simulink model "EKF_MDL"  (R2013a)
settings: Solver=VariableStepDiscrete  StartTime=0.0  StopTime=50  RelTol=1e-3
settings Model: Creator=Aleksandr  LastModifiedBy=Aleksandr

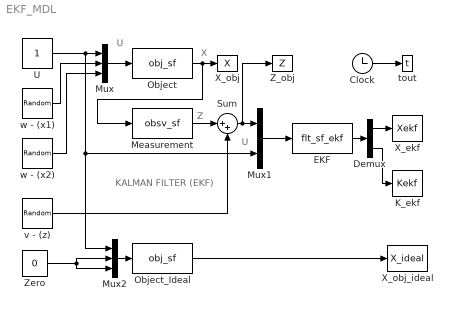
== system EKF_MDL ==
  note: KALMAN FILTER
      | (EKF)
  note: U
  note: Z
  note: U
  note: X
  Clock : Clock
      settings: Decimation=100
  Demux : Demux  Outputs=2
  EKF : S-Function  FunctionName=flt_sf_ekf  EnableBusSupport=off
  K_ekf : ToWorkspace  VariableName=Kekf  SampleTime=-1
  Measurement : S-Function  FunctionName=obsv_sf  EnableBusSupport=off
  Mux : Mux  Inputs=3
  Mux1 : Mux  Inputs=2
  Mux2 : Mux  Inputs=3
  Object : S-Function  FunctionName=obj_sf  EnableBusSupport=off
  Object_Ideal : S-Function  FunctionName=obj_sf  EnableBusSupport=off
  Sum : Sum  Inputs=|++
  U : Constant
  X_ekf : ToWorkspace  VariableName=Xekf  SampleTime=-1
  X_obj : ToWorkspace  VariableName=X  SampleTime=-1
  X_obj_ideal : ToWorkspace  VariableName=X_ideal  SampleTime=-1
  Z_obj : ToWorkspace  VariableName=Z  SampleTime=-1
  Zero : Constant  Value=0
  tout : ToWorkspace  VariableName=t  SampleTime=-1
  v - (z) : RandomNumber  Variance=1.15  SampleTime=0.1
  w - (x1) : RandomNumber  Variance=0.01  SampleTime=0.1
  w - (x2) : RandomNumber  Variance=0.04  SampleTime=0.1
  wires:
  Mux/1 -> Object/1
  w - (x2)/1 -> Mux/3
  w - (x1)/1 -> Mux/2
  Measurement/1 -> Sum/1
  v - (z)/1 -> Sum/2
  Mux1/1 -> EKF/1
  Sum/1 -> Z_obj/1, Mux1/1
  U/1 -> Mux2/1, Mux1/2, Mux/1
  Clock/1 -> tout/1
  Object_Ideal/1 -> X_obj_ideal/1
  Mux2/1 -> Object_Ideal/1
  Zero/1 -> Mux2/2, Mux2/3
  Object/1 -> Measurement/1, X_obj/1
  EKF/1 -> Demux/1
  Demux/1 -> X_ekf/1
  Demux/2 -> K_ekf/1
